simulink library "csc_stg_tracker_sensor_prep_lib"  (R2014b)
settings: Solver=ode45  SolverMode=SingleTasking  StartTime=0.0  StopTime=10.0  RelTol=1e-3
values from neighbouring files (symbols this model uses):
  snp_stg_index = [4 5 6]    [csc_snp_sensor_prep_init.m]
  snp_stg_zero_index = [0 0 0]    [csc_snp_sensor_prep_init.m]
undefined symbols (not defined in the file or in its folder): kfl_use_tracker_meas, stg_body_to_head1
libraries: util_quat_lib x6, util_info_lib x1, csu_und_unduplicate_lib x1, util_common_lib x1
settings Model: ExtModeAutoUpdateStatusClock=off  Creator=Administrator  LastModifiedBy=mstewart

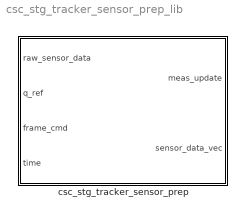
== system csc_stg_tracker_sensor_prep_lib ==
  csc_stg_tracker_sensor_prep : Subsystem

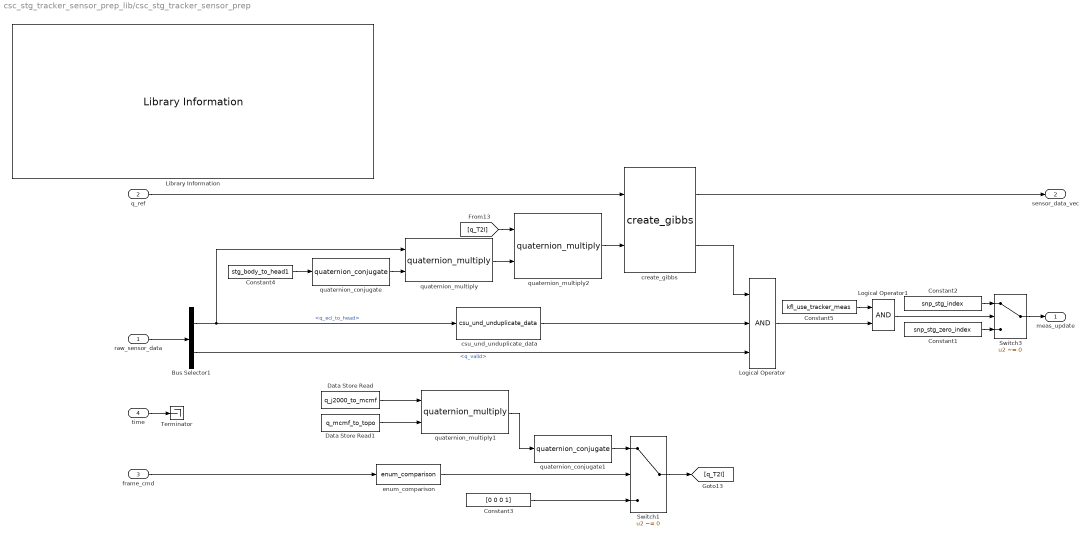
== system csc_stg_tracker_sensor_prep_lib/csc_stg_tracker_sensor_prep ==
  raw_sensor_data : Inport
  q_ref : Inport  Port=2
  frame_cmd : Inport  Port=3
  time : Inport  Port=4
  Bus Selector1 : BusSelector  OutputSignals=q_eci_to_head,q_valid
  Constant1 : Constant  Value=snp_stg_zero_index
  Constant2 : Constant  Value=snp_stg_index
  Constant3 : Constant  Value=[0 0 0 1]
  Constant4 : Constant  Value=stg_body_to_head1
  Constant5 : Constant  Value=kfl_use_tracker_meas
  Data Store Read : DataStoreRead  DataStoreName=q_j2000_to_mcmf
  Data Store Read1 : DataStoreRead  DataStoreName=q_mcmf_to_topo
  Library Information : util_info_lib/Library Information  owner='NONE'
  Logical Operator : Logic  Inputs=3  AllPortsSameDT=off  OutDataTypeStr=boolean
  Logical Operator1 : Logic  AllPortsSameDT=off  OutDataTypeStr=boolean
  Switch1 : Switch  Criteria=u2 ~= 0
  Switch3 : Switch  Criteria=u2 ~= 0
  Terminator : Terminator
  create_gibbs : util_quat_lib/create_gibbs  SystemSampleTime=-1
  csu_und_unduplicate_data : csu_und_unduplicate_lib/csu_und_unduplicate_data  initial_compare=0
  enum_comparison : util_common_lib/enum_comparison  comparison_type===
  quaternion_conjugate : util_quat_lib/quaternion_conjugate  SystemSampleTime=-1
  quaternion_conjugate1 : util_quat_lib/quaternion_conjugate  SystemSampleTime=-1
  quaternion_multiply : util_quat_lib/quaternion_multiply  SystemSampleTime=-1
  quaternion_multiply1 : util_quat_lib/quaternion_multiply  SystemSampleTime=-1
  quaternion_multiply2 : util_quat_lib/quaternion_multiply  SystemSampleTime=-1
  meas_update : Outport
  sensor_data_vec : Outport  Port=2
  wires:
  Data Store Read1/1 -> quaternion_multiply1/2
  Data Store Read/1 -> quaternion_multiply1/1
  Logical Operator1/1 -> Switch3/2
  Constant5/1 -> Logical Operator1/1
  Logical Operator/1 -> Logical Operator1/2
  quaternion_conjugate1/1 -> Switch1/1
  quaternion_multiply2/1 -> create_gibbs/2
  [q_T2I] -> quaternion_multiply2/1
  quaternion_multiply/1 -> quaternion_multiply2/2
  Switch1/1 -> [q_T2I]
  time/1 -> Terminator/1
  quaternion_multiply1/1 -> quaternion_conjugate1/1
  Constant3/1 -> Switch1/3
  enum_comparison/1 -> Switch1/2
  frame_cmd/1 -> enum_comparison/1
  q_ref/1 -> create_gibbs/1
  create_gibbs/1 -> sensor_data_vec/1
  quaternion_conjugate/1 -> quaternion_multiply/2
  Constant4/1 -> quaternion_conjugate/1
  create_gibbs/2 -> Logical Operator/1
  csu_und_unduplicate_data/1 -> Logical Operator/2
  Bus Selector1/2 -> Logical Operator/3  "<q_valid>"
  raw_sensor_data/1 -> Bus Selector1/1
  Bus Selector1/1 -> quaternion_multiply/1, csu_und_unduplicate_data/1  "<q_eci_to_head>"
  Switch3/1 -> meas_update/1
  Constant2/1 -> Switch3/1
  Constant1/1 -> Switch3/3
